simulink subsystem "PieroModelo"  (R2023b)
settings: Solver=VariableStepAuto  StartTime=0.0  StopTime=10.0  RelTol=1e-3
settings Model: Creator=chaya  LastModifiedBy=Pablo

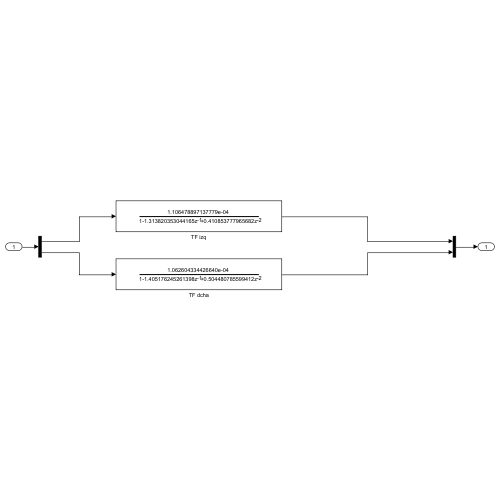
[thumbnail: Simulink's stored preview of the top-level diagram]
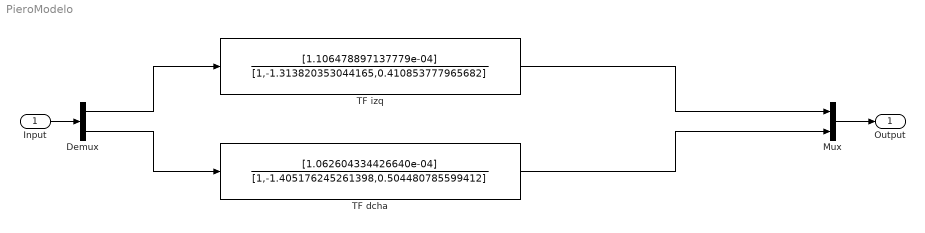
== system PieroModelo ==
  Input : Inport
  Demux : Demux  Outputs=2
  Mux : Mux  Inputs=2
  TF dcha : DiscreteFilter  Numerator=[1.062604334426640e-04]  Denominator=[1,-1.405176245261398,0.504480785599412]
  TF izq : DiscreteFilter  Numerator=[1.106478897137779e-04]  Denominator=[1,-1.313820353044165,0.410853777965682]
  Output : Outport
  wires:
  Input/1 -> Demux/1
  Mux/1 -> Output/1
  Demux/1 -> TF izq/1
  Demux/2 -> TF dcha/1
  TF izq/1 -> Mux/1
  TF dcha/1 -> Mux/2
